simulink model "ex1"  (R2018a)
settings: Solver=VariableStepAuto  StartTime=0.0  StopTime=60  RelTol=1e-5
settings Model: Creator=HUAWEI  LastModifiedBy=HUAWEI

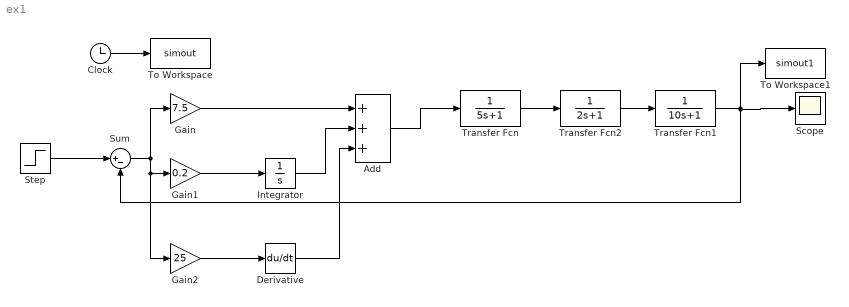
== system ex1 ==
  Add : Sum  Inputs=3
  Clock : Clock
  Derivative : Derivative
  Gain : Gain  Gain=7.5
  Gain1 : Gain  Gain=0.2
  Gain2 : Gain  Gain=25
  Integrator : Integrator
  Scope : Scope
  Step : Step  SampleTime=0
  Sum : Sum  Inputs=|+-
  To Workspace : ToWorkspace  VariableName=simout  SaveFormat=Timeseries  SampleTime=-1
  To Workspace1 : ToWorkspace  VariableName=simout1  SaveFormat=Timeseries  SampleTime=-1
  Transfer Fcn : TransferFcn  Denominator=[5 1]
  Transfer Fcn1 : TransferFcn  Denominator=[10 1]
  Transfer Fcn2 : TransferFcn  Denominator=[2 1]
  wires:
  Step/1 -> Sum/1
  Clock/1 -> To Workspace/1
  Transfer Fcn2/1 -> Transfer Fcn1/1
  Add/1 -> Transfer Fcn/1
  Transfer Fcn/1 -> Transfer Fcn2/1
  Gain/1 -> Add/1
  Integrator/1 -> Add/2
  Derivative/1 -> Add/3
  Gain1/1 -> Integrator/1
  Gain2/1 -> Derivative/1
  Sum/1 -> Gain2/1, Gain1/1, Gain/1
  Transfer Fcn1/1 -> Scope/1, Sum/2, To Workspace1/1
